simulink subsystem "AnalogInputFiltering"  (R2019b)
settings: Solver=VariableStepAuto  StartTime=0.0  StopTime=10.0  RelTol=1e-3
undefined symbols (not defined in the file): motorCurrZero_mV, throttlePos1Max_cnt, throttlePos1Min_cnt, throttlePos2Max_cnt, throttlePos2Min_cnt
libraries: dspstat3 x2, eeGeneralControl x1
settings Model: Creator=Nick  LastModifiedBy=Nick

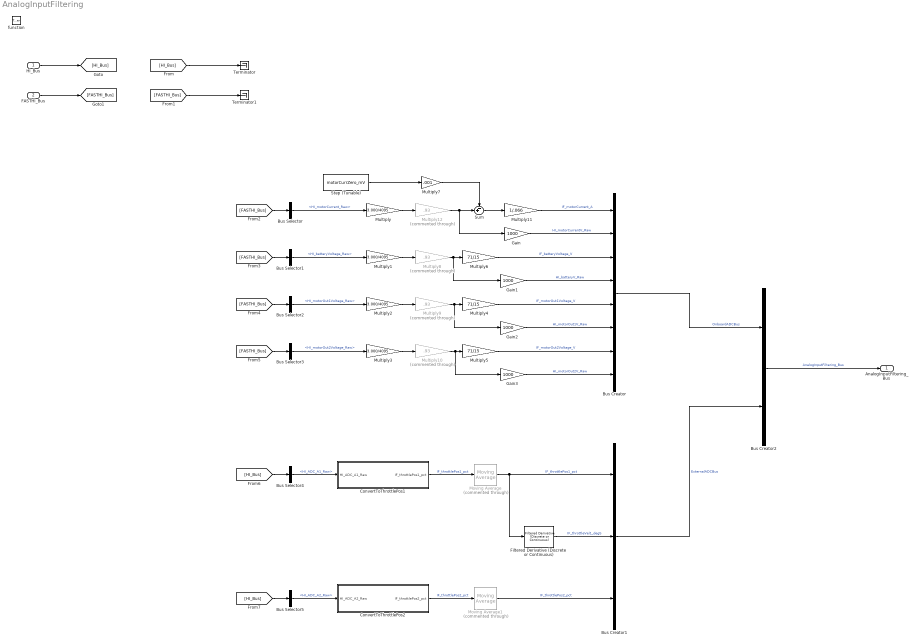
== system AnalogInputFiltering ==
  HI_Bus : Inport
  FASTHI_Bus : Inport  Port=2
  function : TriggerPort  TriggerType=function-call  VariantControl=Variant
  Bus Creator : BusCreator  Inputs=8
  Bus Creator1 : BusCreator  Inputs=3
  Bus Creator2 : BusCreator  Inputs=2
  Bus Selector : BusSelector  OutputSignals=HI_motorCurrent_Raw
  Bus Selector1 : BusSelector  OutputSignals=HI_batteryVoltage_Raw
  Bus Selector2 : BusSelector  OutputSignals=HI_motorOut1Voltage_Raw
  Bus Selector3 : BusSelector  OutputSignals=HI_motorOut2Voltage_Raw
  Bus Selector4 : BusSelector  OutputSignals=SPIBus.HI_ADC_A1_Raw
  Bus Selector5 : BusSelector  OutputSignals=SPIBus.HI_ADC_A2_Raw
  ConvertToThrottlePos1 : Subsystem
  ConvertToThrottlePos2 : Subsystem
  Filtered Derivative (Discrete or Continuous) : eeGeneralControl/Filtered Derivative (Discrete or Continuous)  K=1  T=0.01  B=inf  A=-inf  minRatio=10  Ts=-1
      settings: SourceProductName=Simscape Electrical  SourceProductBaseCode=PS
  Gain{,1..3} (4 alike) : Gain  Gain=1000
  Moving Average : dspstat3/Moving Average  Commented=through  Method=Sliding window  ForgettingFactorPort=off  SpecifyWindowLength=on  WindowLength=10  ForgettingFactor=0.9  SimulateUsing=Code generation
  Moving Average1 : dspstat3/Moving Average  Commented=through  Method=Sliding window  ForgettingFactorPort=off  SpecifyWindowLength=on  WindowLength=10  ForgettingFactor=0.9  SimulateUsing=Code generation
  Multiply{,1..3} (4 alike) : Gain  Gain=3.000/4095
  Multiply{8..10,12} (4 alike) : Gain  Commented=through  Gain=.93
  Multiply11 : Gain  Gain=1/.066
  Multiply4 : Gain  Gain=71/15
  Multiply5 : Gain  Gain=71/15
  Multiply6 : Gain  Gain=71/15
  Multiply7 : Gain  Gain=.001
  Step (Tunable) : Constant  Value=motorCurrZero_mV  VectorParams1D=off  SampleTime=-1
  Sum : Sum  Inputs=-+|
  Terminator : Terminator
  Terminator1 : Terminator
  AnalogInputFiltering_Bus : Outport
  wires:
  Moving Average1/1 -> Bus Creator1/3  "IF_throttlePos2_pct"
  Moving Average/1 -> Filtered Derivative (Discrete or Continuous)/1, Bus Creator1/1  "IF_throttlePos1_pct"
  Step (Tunable)/1 -> Multiply7/1
  [HI_Bus] -> Bus Selector5/1
  Bus Creator1/1 -> Bus Creator2/2  "ExternalADCBus"
  Bus Creator/1 -> Bus Creator2/1  "OnboardADCBus"
  [HI_Bus] -> Bus Selector4/1
  Bus Creator2/1 -> AnalogInputFiltering_Bus/1  "AnalogInputFiltering_Bus"
  HI_Bus/1 -> [HI_Bus]
  [HI_Bus] -> Terminator/1
  [FASTHI_Bus] -> Terminator1/1
  FASTHI_Bus/1 -> [FASTHI_Bus]
  Multiply12/1 -> Sum/2, Gain/1
  Multiply5/1 -> Bus Creator/7  "IF_motorOut2Voltage_V"
  Multiply9/1 -> Multiply4/1, Gain2/1
  Multiply3/1 -> Multiply10/1
  Multiply10/1 -> Multiply5/1, Gain3/1
  Multiply7/1 -> Sum/1
  Multiply6/1 -> Bus Creator/3  "IF_batteryVoltage_V"
  Multiply2/1 -> Multiply9/1
  Multiply/1 -> Multiply12/1
  Multiply8/1 -> Multiply6/1, Gain1/1
  Multiply4/1 -> Bus Creator/5  "IF_motorOut1Voltage_V"
  Multiply1/1 -> Multiply8/1
  Sum/1 -> Multiply11/1
  Multiply11/1 -> Bus Creator/1  "IF_motorCurrent_A"
  Bus Selector3/1 -> Multiply3/1  "<HI_motorOut2Voltage_Raw>"
  Bus Selector2/1 -> Multiply2/1  "<HI_motorOut1Voltage_Raw>"
  Bus Selector1/1 -> Multiply1/1  "<HI_batteryVoltage_Raw>"
  Bus Selector/1 -> Multiply/1  "<HI_motorCurrent_Raw>"
  [FASTHI_Bus] -> Bus Selector/1
  [FASTHI_Bus] -> Bus Selector3/1
  [FASTHI_Bus] -> Bus Selector2/1
  [FASTHI_Bus] -> Bus Selector1/1
  Bus Selector4/1 -> ConvertToThrottlePos1/1(HI_ADC_A1_Raw)  "<HI_ADC_A1_Raw>"
  ConvertToThrottlePos1/1(IF_throttlePos1_pct) -> Moving Average/1  "IF_throttlePos1_pct"
  Bus Selector5/1 -> ConvertToThrottlePos2/1(HI_ADC_A2_Raw)  "<HI_ADC_A2_Raw>"
  ConvertToThrottlePos2/1(IF_throttlePos2_pct) -> Moving Average1/1  "IF_throttlePos2_pct"
  Gain/1 -> Bus Creator/2  "HI_motorCurrentV_Raw"
  Gain1/1 -> Bus Creator/4  "HI_batteryV_Raw"
  Gain2/1 -> Bus Creator/6  "HI_motorOut1V_Raw"
  Gain3/1 -> Bus Creator/8  "HI_motorOut2V_Raw"
  Filtered Derivative (Discrete or Continuous)/1 -> Bus Creator1/2  "IF_throttleVel1_degS"

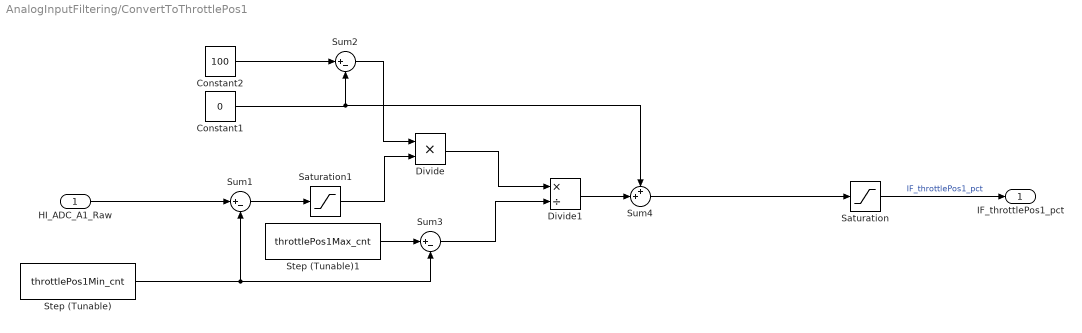
== system AnalogInputFiltering/ConvertToThrottlePos1 ==
  HI_ADC_A1_Raw : Inport
  Constant1 : Constant  Value=0
  Constant2 : Constant  Value=100
  Divide : Product  Inputs=**
  Divide1 : Product  Inputs=*/
  Saturation : Saturate  UpperLimit=100  LowerLimit=0
  Saturation1 : Saturate  UpperLimit=4095  LowerLimit=0
  Step (Tunable) : Constant  Value=throttlePos1Min_cnt  VectorParams1D=off  SampleTime=-1
  Step (Tunable)1 : Constant  Value=throttlePos1Max_cnt  VectorParams1D=off  SampleTime=-1
  Sum1 : Sum  Inputs=|+-
  Sum2 : Sum  Inputs=|+-
  Sum3 : Sum  Inputs=|+-
  Sum4 : Sum  Inputs=++|
  IF_throttlePos1_pct : Outport
  wires:
  Saturation1/1 -> Divide/2
  Saturation/1 -> IF_throttlePos1_pct/1  "IF_throttlePos1_pct"
  HI_ADC_A1_Raw/1 -> Sum1/1
  Constant2/1 -> Sum2/1
  Divide/1 -> Divide1/1
  Sum2/1 -> Divide/1
  Sum1/1 -> Saturation1/1
  Divide1/1 -> Sum4/2
  Sum3/1 -> Divide1/2
  Step (Tunable)/1 -> Sum3/2, Sum1/2
  Constant1/1 -> Sum2/2, Sum4/1
  Sum4/1 -> Saturation/1
  Step (Tunable)1/1 -> Sum3/1

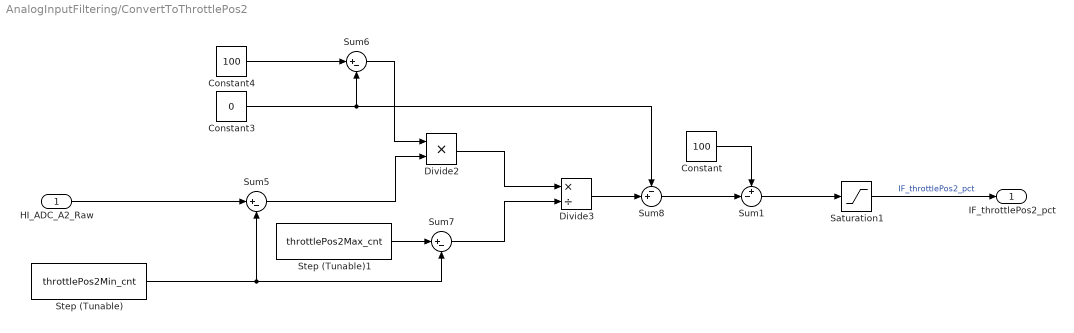
== system AnalogInputFiltering/ConvertToThrottlePos2 ==
  HI_ADC_A2_Raw : Inport
  Constant : Constant  Value=100
  Constant3 : Constant  Value=0
  Constant4 : Constant  Value=100
  Divide2 : Product  Inputs=**
  Divide3 : Product  Inputs=*/
  Saturation1 : Saturate  UpperLimit=100  LowerLimit=0
  Step (Tunable) : Constant  Value=throttlePos2Min_cnt  VectorParams1D=off  SampleTime=-1
  Step (Tunable)1 : Constant  Value=throttlePos2Max_cnt  VectorParams1D=off  SampleTime=-1
  Sum1 : Sum  Inputs=+-|
  Sum5 : Sum  Inputs=|+-
  Sum6 : Sum  Inputs=|+-
  Sum7 : Sum  Inputs=|+-
  Sum8 : Sum  Inputs=-+|
  IF_throttlePos2_pct : Outport
  wires:
  Saturation1/1 -> IF_throttlePos2_pct/1  "IF_throttlePos2_pct"
  Step (Tunable)1/1 -> Sum7/1
  Divide2/1 -> Divide3/1
  Sum7/1 -> Divide3/2
  Constant4/1 -> Sum6/1
  Constant3/1 -> Sum8/1, Sum6/2
  Sum5/1 -> Divide2/2
  Sum6/1 -> Divide2/1
  Sum8/1 -> Sum1/2
  Divide3/1 -> Sum8/2
  Step (Tunable)/1 -> Sum7/2, Sum5/2
  HI_ADC_A2_Raw/1 -> Sum5/1
  Sum1/1 -> Saturation1/1
  Constant/1 -> Sum1/1
